simulink model "Katex_FullCar_R2017b_V03"  (R2026a)
settings: Solver=ode1  StopTime=1000  FixedStep=Ts  EnableMultiTasking=on
PostLoadFcn:
  | , if any(exist('dsrtsu_mdlpostloadfcn', 'file') == [2, 3, 6]), try dsrtsu_mdlpostloadfcn('Execute', bdroot); catch fprintf('Error in PostLoadFcn (dsrtsu_mdlpostloadfcn) for model "%s":\n %s\n', bdroot, lasterr); end, end,
  | , if any(exist('dsrtsu_mdlpostloadfcn', 'file') ~= 0), dsrtsu_mdlpostloadfcn('Execute', bdroot); end,
InitFcn:
  | , if any(exist('rtifpga_mdlclblib', 'file') ~= 0), rtifpga_mdlclblib('Init', bdroot); end,
  | 
  | 
  | init
undefined symbols (not defined in the file): locklim_sus, roundN, Ts
libraries: sl_discontinuities x29, simulink_extras x26, simulink x22, mjLib x1
(part 6 of 10)

== system Katex_FullCar_R2017b_V03/DGIST/_High_Level_Ctrl/Chassis_FB_ctrl/Slip control FR/Subsystem/Subsystem1 ==
  In1 : Inport
  Constant2 : Constant
  Constant3 : Constant  Value=-1
  If : If  IfExpression=u1 >= 0  ElseIfExpressions=u1<0
  If Action Subsystem : Subsystem  TreatAsAtomicUnit=on
  If Action Subsystem1 : Subsystem  TreatAsAtomicUnit=on
  Merge : Merge
  sign : Outport  VectorParamsAs1DForOutWhenUnconnected=off
  wires:
  If Action Subsystem/1(Out1) -> Merge/1
  If Action Subsystem1/1(Out1) -> Merge/2
  Constant3/1 -> If Action Subsystem1/1(In1)
  In1/1 -> If/1
  Merge/1 -> sign/1
  Constant2/1 -> If Action Subsystem/1(In1)
  If/2 -> If Action Subsystem1/Action
  If/1 -> If Action Subsystem/Action

== system Katex_FullCar_R2017b_V03/DGIST/_Low_Level_Ctrl/Driving_Low_Level_Controller/Torque Mode/Driving Wheel Control/DOB(omega) ==
  U_in*(Tm) : Inport
  Y_out(w) : Inport  Port=2
  CutoffFreq_Q : Inport  Port=3
  ControlOnOff : Inport  Port=4
  Add1 : Sum  Inputs=-+
  Add2 : Sum  Inputs=+++
  Delay : Delay  DelayLength=1  InitialCondition=0
  Divide{1..2,4..6} (5 alike) : Product  Inputs=**
  Dot2 : Subsystem
      mask Display: disp('dot')
  LPF : Subsystem
  Dist_hat : Outport  VectorParamsAs1DForOutWhenUnconnected=off
  wires:
  Add1/1 -> LPF/1(In)
  CutoffFreq_Q/1 -> LPF/2(fc)
  LPF/1(Out) -> Divide6/1
  Dot2/1(out) -> Divide2/2
  ControlOnOff/1 -> Divide6/2, Divide5/2, Divide1/2
  Y_out(w)/1 -> Divide1/1
  [Local_Bn] -> Divide4/1
  Divide2/1 -> Add2/1
  [Local_Jn] -> Divide2/1
  Divide1/1 -> Divide4/2, Dot2/1(in)
  Divide4/1 -> Add2/2
  Add2/1 -> Add1/2
  U_in*(Tm)/1 -> Delay/1
  Divide5/1 -> Add1/1
  Divide6/1 -> Dist_hat/1
  [wheel_Bn] -> [Local_Bn]
  [wheel_Jn] -> [Local_Jn]
  Delay/1 -> Divide5/1

== system Katex_FullCar_R2017b_V03/DGIST/_Low_Level_Ctrl/Driving_Low_Level_Controller/Torque Mode/Driving Wheel Control/Feedforward(omega) ==
  command : Inport
  LFP cutoff : Inport  Port=2
  ControlOnOff : Inport  Port=3
  Add5 : Sum  Inputs=+++
  Divide{,1..2,4} (4 alike) : Product  Inputs=**
  Dot2 : Subsystem
      mask Display: disp('dot')
  LPF : Subsystem
  FF : Outport  VectorParamsAs1DForOutWhenUnconnected=off
  wires:
  LFP cutoff/1 -> LPF/2(fc)
  Add5/1 -> LPF/1(In)
  LPF/1(Out) -> Divide/1
  Divide/1 -> FF/1
  ControlOnOff/1 -> Divide1/2, Divide/2
  Divide1/1 -> Divide4/2, Dot2/1(in)
  [wheel_Jn] -> [Local_Jn]
  [wheel_Bn] -> [Local_Bn]
  command/1 -> Divide1/1
  Divide2/1 -> Add5/1
  Dot2/1(out) -> Divide2/2
  [Local_Jn] -> Divide2/1
  Divide4/1 -> Add5/2
  [Local_Bn] -> Divide4/1

== system Katex_FullCar_R2017b_V03/DGIST/_Low_Level_Ctrl/Driving_Low_Level_Controller/Torque Mode/Driving Wheel Control/Poleplacement(PI)1 ==
  note: H(s) = (Kp+Ki)/(s)
  error : Inport
  BW : Inport  Port=2
  zeta : Inport  Port=3
  ConstrolOnOff : Inport  Port=4
  ControlInputError : Inport  Port=5
  Add : Sum
  Add1 : Sum  Inputs=+-
  Constant1 : Constant  Value=Ts
  Divide{,1..5,7} (7 alike) : Product  Inputs=**
  Divide6 : Product  Inputs=***
  Divide9 : Product  Inputs=**/
  Integrator1 : Subsystem
      mask Display: disp('Integator')
  Saturation : Saturate  UpperLimit=3  LowerLimit=0.5
  Saturation Dynamic : sl_discontinuities/Saturation Dynamic  OutMin=[]  OutMax=[]  OutDataTypeStr=Inherit: Same as second input  OutDataType=fixdt(1, 16)  OutScaling=2^-10  DoSatur=off
  Sum1 : Sum  Inputs=|++
  Sum2 : Sum  Inputs=++|
  "gain " : Gain  Gain=2*pi
  gain 1 : Gain  Gain=2
  feedback gain : Outport  VectorParamsAs1DForOutWhenUnconnected=off
  wires:
  BW/1 -> "gain "/1
  zeta/1 -> Saturation/1
  Saturation/1 -> gain 1/1
  [Local_Bn] -> Add1/2
  Divide1/1 -> Sum1/1
  Divide2/1 -> Sum1/2
  Integrator1/1(out) -> Divide2/1
  gain 1/1 -> Divide6/1
  Divide3/1 -> Divide4/1
  [wheel_Bn] -> [Local_Bn]
  [wheel_Jn] -> [Local_Jn]
  [Local_Jn] -> Divide4/2
  [Local_Jn] -> Divide6/3
  Divide6/1 -> Add1/1
  Add1/1 -> [Kp]
  Divide4/1 -> [Ki]
  [Kp] -> Divide1/1
  error/1 -> Divide/1
  Sum1/1 -> Divide5/1
  Divide5/1 -> feedback gain/1
  ConstrolOnOff/1 -> Divide5/2, Integrator1/2("Off : 0 On : 1"), Divide/2
  [Ki] -> Divide2/2
  ControlInputError/1 -> Divide7/1
  Divide/1 -> Divide1/2, Sum2/1
  Sum2/1 -> Integrator1/1(in)
  Divide7/1 -> Sum2/2
  Add/1 -> Saturation Dynamic/1
  Divide9/1 -> [AntiWindup]
  Constant1/1 -> Saturation Dynamic/3
  "gain "/1 -> Divide9/2, Add/1, Divide9/1, Divide6/2, Divide3/1, Divide3/2
  [Ki] -> Add/2, Saturation Dynamic/2
  [AntiWindup] -> Divide7/2
  Saturation Dynamic/1 -> Divide9/3

== system Katex_FullCar_R2017b_V03/DGIST/_Low_Level_Ctrl/Driving_Low_Level_Controller/Torque Mode/Driving Wheel Control/Subsystem ==
  note: wheel N*m
  note: mN*m
  note: Motor N*m
  N*m : Inport
  Constant1 : Constant  Value=1000
  Divide : Product  Inputs=*/
  Divide1 : Product  Inputs=**
  Divide3 : Product  Inputs=*/
  Gain : Gain  Gain=1000
  Gain1 : Gain  Gain=-1
  Saturation Dynamic : sl_discontinuities/Saturation Dynamic  OutMin=[]  OutMax=[]  OutDataTypeStr=Inherit: Same as second input  OutDataType=fixdt(1, 16)  OutScaling=2^-10  DoSatur=off
  Target Torque : Outport  VectorParamsAs1DForOutWhenUnconnected=off
  wires:
  [N_dri] -> Divide3/2
  Gain/1 -> Target Torque/1
  Divide/1 -> Gain/1
  N*m/1 -> Divide3/1
  Divide1/1 -> Saturation Dynamic/2
  Constant1/1 -> Divide1/2
  Divide3/1 -> Divide1/1
  Saturation Dynamic/1 -> Divide/1
  Gain1/1 -> Saturation Dynamic/3
  [Dri_rated_torque] -> Saturation Dynamic/1, Gain1/1, Divide/2

== system Katex_FullCar_R2017b_V03/DGIST/_Low_Level_Ctrl/Steering_Low_Level_Controller/Torque Mode/Steering Motor Control/DOB(omega) ==
  U_in*(Tm) : Inport
  Y_out(w) : Inport  Port=2
  CutoffFreq_Q : Inport  Port=3
  ControlOnOff : Inport  Port=4
  Add1 : Sum  Inputs=-+
  Add2 : Sum  Inputs=+++
  Delay : Delay  DelayLength=1  InitialCondition=0
  Divide{1..2,4..6} (5 alike) : Product  Inputs=**
  Dot2 : Subsystem
      mask Display: disp('dot')
  LPF : Subsystem
  Dist_hat : Outport  VectorParamsAs1DForOutWhenUnconnected=off
  wires:
  Add1/1 -> LPF/1(In)
  CutoffFreq_Q/1 -> LPF/2(fc)
  LPF/1(Out) -> Divide6/1
  Dot2/1(out) -> Divide2/2
  ControlOnOff/1 -> Divide6/2, Divide5/2, Divide1/2
  Y_out(w)/1 -> Divide1/1
  [Local_Bn] -> Divide4/1
  Divide2/1 -> Add2/1
  [Local_Jn] -> Divide2/1
  Divide1/1 -> Divide4/2, Dot2/1(in)
  Divide4/1 -> Add2/2
  Add2/1 -> Add1/2
  U_in*(Tm)/1 -> Delay/1
  Divide5/1 -> Add1/1
  Divide6/1 -> Dist_hat/1
  [steer_Bn] -> [Local_Bn]
  [steer_Jn] -> [Local_Jn]
  Delay/1 -> Divide5/1

== system Katex_FullCar_R2017b_V03/DGIST/_Low_Level_Ctrl/Steering_Low_Level_Controller/Torque Mode/Steering Motor Control/DOB(theta) ==
  U_in*(Tm) : Inport
  Y_out(theta) : Inport  Port=2
  CutoffFreq_Q : Inport  Port=3
  ConstrolOnOff : Inport  Port=4
  Add1 : Sum  Inputs=-+
  Add5 : Sum  Inputs=+++
  Delay : Delay  DelayLength=1  InitialCondition=0
  Divide{,1..5} (6 alike) : Product  Inputs=**
  Dot : Subsystem
      mask Display: disp('dot')
  Dot1 : Subsystem
      mask Display: disp('dot')
  Dot2 : Subsystem
      mask Display: disp('dot')
  NominalModel_Kn : Constant  Value=0
  Scope1 : Scope
  Scope2 : Scope
      settings: DataLoggingVariableName=ScopeData2
  Scope3 : Scope
      settings: DataLoggingVariableName=ScopeData3
  Second order LPF : Subsystem
  zeta : Constant  SampleTime=Ts
  Dist_hat : Outport  VectorParamsAs1DForOutWhenUnconnected=off
  wires:
  Add5/1 -> Add1/2
  CutoffFreq_Q/1 -> Second order LPF/2(fc)
  zeta/1 -> Second order LPF/3(zeta)
  [steer_Jn] -> [Local_Jn]
  NominalModel_Kn/1 -> [Local_Kn]
  [steer_Bn] -> [Local_Bn]
  Y_out(theta)/1 -> Scope1/1, Divide4/1
  [Local_Jn] -> Divide/2
  [Local_Kn] -> Divide2/2
  Dot1/1(out) -> Divide1/1
  [Local_Bn] -> Divide1/2
  Dot/1(out) -> Dot2/1(in)
  Divide/1 -> Add5/1
  Divide2/1 -> Add5/3
  Divide1/1 -> Add5/2
  Dot2/1(out) -> Divide/1
  ConstrolOnOff/1 -> Divide5/2, Divide3/2, Divide4/2
  Divide4/1 -> Divide2/1, Dot1/1(in), Dot/1(in)
  U_in*(Tm)/1 -> Delay/1
  Divide3/1 -> Add1/1
  Second order LPF/1(Dist_hat) -> Divide5/1
  Divide5/1 -> Scope2/1, Dist_hat/1
  Delay/1 -> Divide3/1
  Add1/1 -> Scope3/1, Second order LPF/1(In)

== system Katex_FullCar_R2017b_V03/DGIST/_Low_Level_Ctrl/Steering_Low_Level_Controller/Torque Mode/Steering Motor Control/Feedforward(omega) ==
  command : Inport
  LFP cutoff : Inport  Port=2
  ControlOnOff : Inport  Port=3
  Add5 : Sum  Inputs=+++
  Divide{,1..2,4} (4 alike) : Product  Inputs=**
  Dot2 : Subsystem
      mask Display: disp('dot')
  LPF : Subsystem
  FF : Outport  VectorParamsAs1DForOutWhenUnconnected=off
  wires:
  LFP cutoff/1 -> LPF/2(fc)
  Add5/1 -> LPF/1(In)
  LPF/1(Out) -> Divide/1
  Divide/1 -> FF/1
  ControlOnOff/1 -> Divide/2, Divide1/2
  Divide1/1 -> Divide4/2, Dot2/1(in)
  [steer_Jn] -> [Local_Jn]
  [steer_Bn] -> [Local_Bn]
  command/1 -> Divide1/1
  Divide2/1 -> Add5/1
  Dot2/1(out) -> Divide2/2
  [Local_Jn] -> Divide2/1
  Divide4/1 -> Add5/2
  [Local_Bn] -> Divide4/1

== system Katex_FullCar_R2017b_V03/DGIST/_Low_Level_Ctrl/Steering_Low_Level_Controller/Torque Mode/Steering Motor Control/Feedforward(theta) ==
  command : Inport
  LFP cutoff : Inport  Port=2
  LPF zeta : Inport  Port=3
  ConstrolOnOff : Inport  Port=4
  Add5 : Sum  Inputs=+++
  Divide{,1..4} (5 alike) : Product  Inputs=**
  Dot : Subsystem
      mask Display: disp('dot')
  Dot1 : Subsystem
      mask Display: disp('dot')
  Dot2 : Subsystem
      mask Display: disp('dot')
  NominalModel_Kn : Constant  Value=0
  Scope : Scope
      settings: ActiveDisplayYMinimum=-1  ActiveDisplayYMaximum=1  DataLoggingVariableName=ScopeData2
  Scope1 : Scope
      settings: ActiveDisplayYMinimum=-1  ActiveDisplayYMaximum=1  DataLoggingVariableName=ScopeData5
  Second order LPF : Subsystem
  before_dot : Scope
      settings: DataLoggingVariableName=ScopeData3
  commad : Scope
      settings: DataLoggingVariableName=ScopeData4
  FF : Outport  VectorParamsAs1DForOutWhenUnconnected=off
  wires:
  Dot/1(out) -> Dot2/1(in)
  Dot1/1(out) -> Divide1/1
  LFP cutoff/1 -> Second order LPF/2(fc)
  Dot2/1(out) -> Divide/1
  Add5/1 -> Second order LPF/1(In)
  LPF zeta/1 -> Second order LPF/3(zeta)
  Divide/1 -> Scope/1, Add5/1
  Divide1/1 -> Scope1/1, Add5/2
  Divide2/1 -> Add5/3
  [Local_Jn] -> Divide/2
  [Local_Bn] -> Divide1/2
  [Local_Kn] -> Divide2/2
  [steer_Jn] -> [Local_Jn]
  [steer_Bn] -> [Local_Bn]
  NominalModel_Kn/1 -> [Local_Kn]
  Second order LPF/1(Out) -> Divide3/1
  Divide3/1 -> FF/1
  ConstrolOnOff/1 -> Divide4/2, Divide3/2
  Divide4/1 -> Divide2/1, Dot1/1(in), before_dot/1, Dot/1(in)
  command/1 -> commad/1, Divide4/1

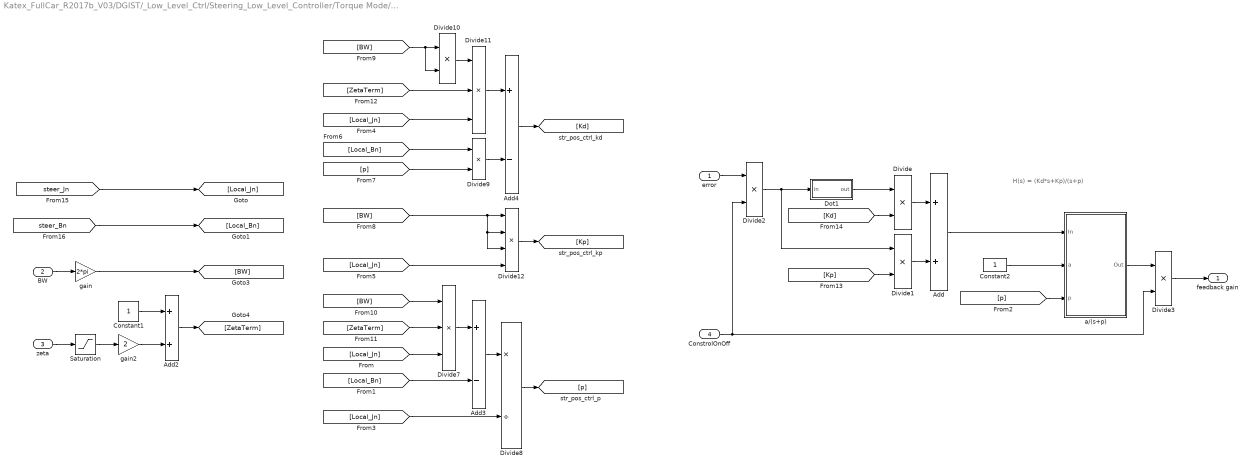
== system Katex_FullCar_R2017b_V03/DGIST/_Low_Level_Ctrl/Steering_Low_Level_Controller/Torque Mode/Steering Motor Control/Lag compensator(zeta) ==
  note: H(s) = (Kd*s+Kp)/(s+p)
  error : Inport
  BW : Inport  Port=2
  zeta : Inport  Port=3
  ConstrolOnOff : Inport  Port=4
  Add : Sum
  Add2 : Sum
  Add3 : Sum  Inputs=+-
  Add4 : Sum  Inputs=+-
  Constant1 : Constant  SampleTime=Ts
  Constant2 : Constant  SampleTime=Ts
  Divide{,1..3,9..10} (6 alike) : Product  Inputs=**
  Divide11 : Product  Inputs=***
  Divide12 : Product  Inputs=****
  Divide7 : Product  Inputs=***
  Divide8 : Product  Inputs=*/
  Dot1 : Subsystem
      mask Display: disp('dot')
  Saturation : Saturate  UpperLimit=1.5  LowerLimit=0.5
  a/(s+p) : Subsystem
  "gain " : Gain  Gain=2*pi
  gain2 : Gain  Gain=2
  feedback gain : Outport  VectorParamsAs1DForOutWhenUnconnected=off
  wires:
  BW/1 -> "gain "/1
  Add/1 -> a/(s+p)/1(In)
  Divide/1 -> Add/1
  Dot1/1(out) -> Divide/1
  Constant2/1 -> a/(s+p)/2(a)
  zeta/1 -> Saturation/1
  Saturation/1 -> gain2/1
  gain2/1 -> Add2/2
  Constant1/1 -> Add2/1
  [Local_Jn] -> Divide7/3
  Divide7/1 -> Add3/1
  [Local_Bn] -> Add3/2
  Add3/1 -> Divide8/1
  Divide10/1 -> Divide11/1
  Divide8/1 -> [p]
  Divide9/1 -> Add4/2
  Divide11/1 -> Add4/1
  [p] -> a/(s+p)/3(p)
  Divide1/1 -> Add/2
  [Local_Jn] -> Divide8/2
  [Local_Jn] -> Divide11/3
  [Local_Jn] -> Divide12/4
  [Local_Bn] -> Divide9/1
  [p] -> Divide9/2
  "gain "/1 -> [BW]
  [BW] -> Divide12/3, Divide12/2, Divide12/1
  [BW] -> Divide10/2, Divide10/1
  [BW] -> Divide7/1
  Add2/1 -> [ZetaTerm]
  [ZetaTerm] -> Divide7/2
  [ZetaTerm] -> Divide11/2
  Add4/1 -> [Kd]
  Divide12/1 -> [Kp]
  [Kp] -> Divide1/2
  [Kd] -> Divide/2
  [steer_Jn] -> [Local_Jn]
  [steer_Bn] -> [Local_Bn]
  error/1 -> Divide2/1
  Divide2/1 -> Divide1/1, Dot1/1(in)
  ConstrolOnOff/1 -> Divide3/2, Divide2/2
  a/(s+p)/1(Out) -> Divide3/1
  Divide3/1 -> feedback gain/1

== system Katex_FullCar_R2017b_V03/DGIST/_Low_Level_Ctrl/Steering_Low_Level_Controller/Torque Mode/Steering Motor Control/Poleplacement(PI)1 ==
  note: H(s) = (Kp+Ki)/(s)
  error : Inport
  BW : Inport  Port=2
  zeta : Inport  Port=3
  ConstrolOnOff : Inport  Port=4
  ControlInputError : Inport  Port=5
  Add : Sum
  Add1 : Sum  Inputs=+-
  Constant1 : Constant  Value=Ts
  Divide{,1..5,7} (7 alike) : Product  Inputs=**
  Divide6 : Product  Inputs=***
  Divide9 : Product  Inputs=**/
  Integrator1 : Subsystem
      mask Display: disp('Integator')
  Saturation : Saturate  UpperLimit=3  LowerLimit=0.5
  Saturation Dynamic : simulink/Discontinuities/Saturation Dynamic  OutMin=[]  OutMax=[]  OutDataTypeStr=Inherit: Same as second input  OutDataType=fixdt(1, 16)  OutScaling=2^-10  DoSatur=off
  Sum1 : Sum  Inputs=|++
  Sum2 : Sum  Inputs=++|
  "gain " : Gain  Gain=2*pi
  gain 1 : Gain  Gain=2
  feedback gain : Outport  VectorParamsAs1DForOutWhenUnconnected=off
  wires:
  BW/1 -> "gain "/1
  zeta/1 -> Saturation/1
  Saturation/1 -> gain 1/1
  [Local_Bn] -> Add1/2
  Divide1/1 -> Sum1/1
  Divide2/1 -> Sum1/2
  Integrator1/1(out) -> Divide2/1
  gain 1/1 -> Divide6/1
  Divide3/1 -> Divide4/1
  [Local_Jn] -> Divide4/2
  [Local_Jn] -> Divide6/3
  Divide6/1 -> Add1/1
  Add1/1 -> [Kp]
  Divide4/1 -> [Ki]
  [Kp] -> Divide1/1
  error/1 -> Divide/1
  Sum1/1 -> Divide5/1
  Divide5/1 -> feedback gain/1
  ConstrolOnOff/1 -> Divide5/2, Integrator1/2("Off : 0 On : 1"), Divide/2
  [Ki] -> Divide2/2
  ControlInputError/1 -> Divide7/1
  Divide/1 -> Divide1/2, Sum2/1
  Sum2/1 -> Integrator1/1(in)
  Divide7/1 -> Sum2/2
  Add/1 -> Saturation Dynamic/1
  Divide9/1 -> [AntiWindup]
  Constant1/1 -> Saturation Dynamic/3
  "gain "/1 -> Divide9/2, Add/1, Divide9/1, Divide6/2, Divide3/1, Divide3/2
  [Ki] -> Add/2, Saturation Dynamic/2
  [AntiWindup] -> Divide7/2
  Saturation Dynamic/1 -> Divide9/3
  [steer_Jn] -> [Local_Jn]
  [steer_Bn] -> [Local_Bn]

== system Katex_FullCar_R2017b_V03/DGIST/_Low_Level_Ctrl/Steering_Low_Level_Controller/Torque Mode/Steering Motor Control/Steering Ref Mode  ==
  Constant2 : Constant  Value=0
  If : If  IfExpression=u1 == 0  ElseIfExpressions=u1 ==1
  If Action Subsystem : Subsystem  TreatAsAtomicUnit=on
  If Action Subsystem1 : Subsystem  TreatAsAtomicUnit=on
  If Action Subsystem2 : Subsystem  TreatAsAtomicUnit=on
  Merge : Merge  Inputs=3
  Out1 : Outport  VectorParamsAs1DForOutWhenUnconnected=off
  wires:
  Constant2/1 -> If Action Subsystem/1(In1)
  [sine_ref] -> If Action Subsystem1/1(In1)
  Merge/1 -> Out1/1
  If Action Subsystem/1(Out1) -> Merge/1
  If Action Subsystem2/1(Out1) -> Merge/3
  [str_load_target_pos] -> If Action Subsystem2/1(In1)
  If Action Subsystem1/1(Out1) -> Merge/2
  If/2 -> If Action Subsystem1/Action
  If/3 -> If Action Subsystem2/Action
  [str_ref_mode] -> If/1
  If/1 -> If Action Subsystem/Action

== system Katex_FullCar_R2017b_V03/DGIST/_Low_Level_Ctrl/Steering_Low_Level_Controller/Torque Mode/Steering Motor Control/Steering system ==
  note: mN*m
  note: Motor N*m
  note: Load N*m
  N*m : Inport
  Constant : Constant  Value=55.08
  Constant1 : Constant  Value=1000
  Constant2 : Constant  Value=315
  Divide : Product  Inputs=*/
  Divide1 : Product  Inputs=**
  Divide3 : Product  Inputs=*/
  Gain : Gain  Gain=1000
  Gain1 : Gain  Gain=-1
  Saturation Dynamic : simulink/Discontinuities/Saturation Dynamic  OutMin=[]  OutMax=[]  OutDataTypeStr=Inherit: Same as second input  OutDataType=fixdt(1, 16)  OutScaling=2^-10  DoSatur=off
  Target Torque : Outport  VectorParamsAs1DForOutWhenUnconnected=off
  tag scope: closed_ID_FB=global
  wires:
  Constant2/1 -> Divide3/2
  Gain/1 -> Target Torque/1
  Divide/1 -> Gain/1
  N*m/1 -> Divide3/1
  Divide1/1 -> [closed_ID_FB], Saturation Dynamic/2
  Constant1/1 -> Divide1/2
  Divide3/1 -> Divide1/1
  Saturation Dynamic/1 -> Divide/1
  Gain1/1 -> Saturation Dynamic/3
  Constant/1 -> Saturation Dynamic/1, Gain1/1, Divide/2

== system Katex_FullCar_R2017b_V03/DGIST/_Low_Level_Ctrl/Steering_Low_Level_Controller/Torque Mode/Steering Motor Control/Steering system1 ==
  note: mN*m
  note: Motor N*m
  note: Load N*m
  N*m : Inport
  Constant1 : Constant  Value=1000
  Constant2 : Constant  Value=315
  Divide : Product  Inputs=*/
  Divide1 : Product  Inputs=**
  Divide3 : Product  Inputs=*/
  Gain : Gain  Gain=1000
  Gain1 : Gain  Gain=-1
  Saturation Dynamic : sl_discontinuities/Saturation Dynamic  OutMin=[]  OutMax=[]  OutDataTypeStr=Inherit: Same as second input  OutDataType=fixdt(1, 16)  OutScaling=2^-10  DoSatur=off
  Target Torque : Outport  VectorParamsAs1DForOutWhenUnconnected=off
  wires:
  Constant2/1 -> Divide3/2
  Gain/1 -> Target Torque/1
  Divide/1 -> Gain/1
  N*m/1 -> Divide3/1
  Divide1/1 -> Saturation Dynamic/2
  Constant1/1 -> Divide1/2
  Divide3/1 -> Divide1/1
  Saturation Dynamic/1 -> Divide/1
  Gain1/1 -> Saturation Dynamic/3
  [str_rated_torque] -> Saturation Dynamic/1, Gain1/1, Divide/2

== system Katex_FullCar_R2017b_V03/DGIST/_Low_Level_Ctrl/Steering_Low_Level_Controller/Torque Mode/Steering Motor Control1/DOB(theta) ==
  U_in*(Tm) : Inport
  Y_out(theta) : Inport  Port=2
  CutoffFreq_Q : Inport  Port=3
  ConstrolOnOff : Inport  Port=4
  Add1 : Sum  Inputs=-+
  Add5 : Sum  Inputs=+++
  Delay : Delay  DelayLength=1  InitialCondition=0
  Divide{,1..5} (6 alike) : Product  Inputs=**
  Dot : Subsystem
      mask Display: disp('dot')
  Dot1 : Subsystem
      mask Display: disp('dot')
  Dot2 : Subsystem
      mask Display: disp('dot')
  NominalModel_Kn : Constant  Value=0
  Scope1 : Scope
  Scope2 : Scope
      settings: DataLoggingVariableName=ScopeData2
  Scope3 : Scope
      settings: DataLoggingVariableName=ScopeData3
  Second order LPF : Subsystem
  zeta : Constant  SampleTime=Ts
  Dist_hat : Outport  VectorParamsAs1DForOutWhenUnconnected=off
  wires:
  Add5/1 -> Add1/2
  CutoffFreq_Q/1 -> Second order LPF/2(fc)
  zeta/1 -> Second order LPF/3(zeta)
  [steer_Jn] -> [Local_Jn]
  NominalModel_Kn/1 -> [Local_Kn]
  [steer_Bn] -> [Local_Bn]
  Y_out(theta)/1 -> Scope1/1, Divide4/1
  [Local_Jn] -> Divide/2
  [Local_Kn] -> Divide2/2
  Dot1/1(out) -> Divide1/1
  [Local_Bn] -> Divide1/2
  Dot/1(out) -> Dot2/1(in)
  Divide/1 -> Add5/1
  Divide2/1 -> Add5/3
  Divide1/1 -> Add5/2
  Dot2/1(out) -> Divide/1
  ConstrolOnOff/1 -> Divide5/2, Divide3/2, Divide4/2
  Divide4/1 -> Divide2/1, Dot1/1(in), Dot/1(in)
  U_in*(Tm)/1 -> Delay/1
  Divide3/1 -> Add1/1
  Second order LPF/1(Dist_hat) -> Divide5/1
  Divide5/1 -> Scope2/1, Dist_hat/1
  Delay/1 -> Divide3/1
  Add1/1 -> Scope3/1, Second order LPF/1(In)

== system Katex_FullCar_R2017b_V03/DGIST/_Low_Level_Ctrl/Steering_Low_Level_Controller/Torque Mode/Steering Motor Control1/Feedforward(theta) ==
  command : Inport
  LFP cutoff : Inport  Port=2
  LPF zeta : Inport  Port=3
  ConstrolOnOff : Inport  Port=4
  Add5 : Sum  Inputs=+++
  Divide{,1..4} (5 alike) : Product  Inputs=**
  Dot : Subsystem
      mask Display: disp('dot')
  Dot1 : Subsystem
      mask Display: disp('dot')
  Dot2 : Subsystem
      mask Display: disp('dot')
  NominalModel_Kn : Constant  Value=0
  Scope : Scope
      settings: ActiveDisplayYMinimum=-1  ActiveDisplayYMaximum=1  DataLoggingVariableName=ScopeData2
  Scope1 : Scope
      settings: ActiveDisplayYMinimum=-1  ActiveDisplayYMaximum=1  DataLoggingVariableName=ScopeData5
  Second order LPF : Subsystem
  before_dot : Scope
      settings: DataLoggingVariableName=ScopeData3
  commad : Scope
      settings: DataLoggingVariableName=ScopeData4
  FF : Outport  VectorParamsAs1DForOutWhenUnconnected=off
  wires:
  Dot/1(out) -> Dot2/1(in)
  Dot1/1(out) -> Divide1/1
  LFP cutoff/1 -> Second order LPF/2(fc)
  Dot2/1(out) -> Divide/1
  Add5/1 -> Second order LPF/1(In)
  LPF zeta/1 -> Second order LPF/3(zeta)
  Divide/1 -> Scope/1, Add5/1
  Divide1/1 -> Scope1/1, Add5/2
  Divide2/1 -> Add5/3
  [Local_Jn] -> Divide/2
  [Local_Bn] -> Divide1/2
  [Local_Kn] -> Divide2/2
  [steer_Jn] -> [Local_Jn]
  [steer_Bn] -> [Local_Bn]
  NominalModel_Kn/1 -> [Local_Kn]
  Second order LPF/1(Out) -> Divide3/1
  Divide3/1 -> FF/1
  ConstrolOnOff/1 -> Divide4/2, Divide3/2
  Divide4/1 -> Divide2/1, Dot1/1(in), before_dot/1, Dot/1(in)
  command/1 -> commad/1, Divide4/1

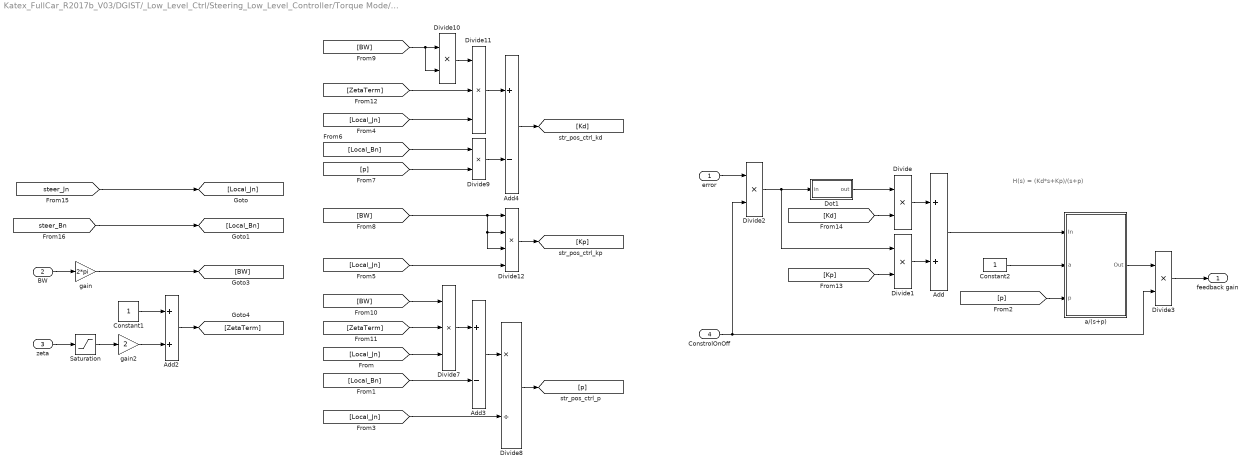
== system Katex_FullCar_R2017b_V03/DGIST/_Low_Level_Ctrl/Steering_Low_Level_Controller/Torque Mode/Steering Motor Control1/Lag compensator(zeta) ==
  note: H(s) = (Kd*s+Kp)/(s+p)
  error : Inport
  BW : Inport  Port=2
  zeta : Inport  Port=3
  ConstrolOnOff : Inport  Port=4
  Add : Sum
  Add2 : Sum
  Add3 : Sum  Inputs=+-
  Add4 : Sum  Inputs=+-
  Constant1 : Constant  SampleTime=Ts
  Constant2 : Constant  SampleTime=Ts
  Divide{,1..3,9..10} (6 alike) : Product  Inputs=**
  Divide11 : Product  Inputs=***
  Divide12 : Product  Inputs=****
  Divide7 : Product  Inputs=***
  Divide8 : Product  Inputs=*/
  Dot1 : Subsystem
      mask Display: disp('dot')
  Saturation : Saturate  UpperLimit=1.5  LowerLimit=0.5
  a/(s+p) : Subsystem
  "gain " : Gain  Gain=2*pi
  gain2 : Gain  Gain=2
  feedback gain : Outport  VectorParamsAs1DForOutWhenUnconnected=off
  wires:
  BW/1 -> "gain "/1
  Add/1 -> a/(s+p)/1(In)
  Divide/1 -> Add/1
  Dot1/1(out) -> Divide/1
  Constant2/1 -> a/(s+p)/2(a)
  zeta/1 -> Saturation/1
  Saturation/1 -> gain2/1
  gain2/1 -> Add2/2
  Constant1/1 -> Add2/1
  [Local_Jn] -> Divide7/3
  Divide7/1 -> Add3/1
  [Local_Bn] -> Add3/2
  Add3/1 -> Divide8/1
  Divide10/1 -> Divide11/1
  Divide8/1 -> [p]
  Divide9/1 -> Add4/2
  Divide11/1 -> Add4/1
  [p] -> a/(s+p)/3(p)
  Divide1/1 -> Add/2
  [Local_Jn] -> Divide8/2
  [Local_Jn] -> Divide11/3
  [Local_Jn] -> Divide12/4
  [Local_Bn] -> Divide9/1
  [p] -> Divide9/2
  "gain "/1 -> [BW]
  [BW] -> Divide12/3, Divide12/2, Divide12/1
  [BW] -> Divide10/2, Divide10/1
  [BW] -> Divide7/1
  Add2/1 -> [ZetaTerm]
  [ZetaTerm] -> Divide7/2
  [ZetaTerm] -> Divide11/2
  Add4/1 -> [Kd]
  Divide12/1 -> [Kp]
  [Kp] -> Divide1/2
  [Kd] -> Divide/2
  [steer_Jn] -> [Local_Jn]
  [steer_Bn] -> [Local_Bn]
  error/1 -> Divide2/1
  Divide2/1 -> Divide1/1, Dot1/1(in)
  ConstrolOnOff/1 -> Divide3/2, Divide2/2
  a/(s+p)/1(Out) -> Divide3/1
  Divide3/1 -> feedback gain/1

== system Katex_FullCar_R2017b_V03/DGIST/_Low_Level_Ctrl/Steering_Low_Level_Controller/Torque Mode/Steering Motor Control1/Steering system1 ==
  note: mN*m
  note: Motor N*m
  note: Load N*m
  N*m : Inport
  Constant1 : Constant  Value=1000
  Constant2 : Constant  Value=315
  Divide : Product  Inputs=*/
  Divide1 : Product  Inputs=**
  Divide3 : Product  Inputs=*/
  Gain : Gain  Gain=1000
  Gain1 : Gain  Gain=-1
  Saturation Dynamic : sl_discontinuities/Saturation Dynamic  OutMin=[]  OutMax=[]  OutDataTypeStr=Inherit: Same as second input  OutDataType=fixdt(1, 16)  OutScaling=2^-10  DoSatur=off
  Target Torque : Outport  VectorParamsAs1DForOutWhenUnconnected=off
  wires:
  Constant2/1 -> Divide3/2
  Gain/1 -> Target Torque/1
  Divide/1 -> Gain/1
  N*m/1 -> Divide3/1
  Divide1/1 -> Saturation Dynamic/2
  Constant1/1 -> Divide1/2
  Divide3/1 -> Divide1/1
  Saturation Dynamic/1 -> Divide/1
  Gain1/1 -> Saturation Dynamic/3
  [str_rated_torque] -> Saturation Dynamic/1, Gain1/1, Divide/2

== system Katex_FullCar_R2017b_V03/DGIST/_Low_Level_Ctrl/Steering_Low_Level_Controller/Torque Mode/Steering Motor Control2/DOB(omega) ==
  U_in*(Tm) : Inport
  Y_out(w) : Inport  Port=2
  CutoffFreq_Q : Inport  Port=3
  ControlOnOff : Inport  Port=4
  Add1 : Sum  Inputs=-+
  Add2 : Sum  Inputs=+++
  Delay : Delay  DelayLength=1  InitialCondition=0
  Divide{1..2,4..6} (5 alike) : Product  Inputs=**
  Dot2 : Subsystem
      mask Display: disp('dot')
  LPF : Subsystem
  Dist_hat : Outport  VectorParamsAs1DForOutWhenUnconnected=off
  wires:
  Add1/1 -> LPF/1(In)
  CutoffFreq_Q/1 -> LPF/2(fc)
  LPF/1(Out) -> Divide6/1
  Dot2/1(out) -> Divide2/2
  ControlOnOff/1 -> Divide6/2, Divide5/2, Divide1/2
  Y_out(w)/1 -> Divide1/1
  [Local_Bn] -> Divide4/1
  Divide2/1 -> Add2/1
  [Local_Jn] -> Divide2/1
  Divide1/1 -> Divide4/2, Dot2/1(in)
  Divide4/1 -> Add2/2
  Add2/1 -> Add1/2
  U_in*(Tm)/1 -> Delay/1
  Divide5/1 -> Add1/1
  Divide6/1 -> Dist_hat/1
  [steer_Bn] -> [Local_Bn]
  [steer_Jn] -> [Local_Jn]
  Delay/1 -> Divide5/1

== system Katex_FullCar_R2017b_V03/DGIST/_Low_Level_Ctrl/Steering_Low_Level_Controller/Torque Mode/Steering Motor Control2/DOB(theta) ==
  U_in*(Tm) : Inport
  Y_out(theta) : Inport  Port=2
  CutoffFreq_Q : Inport  Port=3
  ConstrolOnOff : Inport  Port=4
  Add1 : Sum  Inputs=-+
  Add5 : Sum  Inputs=+++
  Delay : Delay  DelayLength=1  InitialCondition=0
  Divide{,1..5} (6 alike) : Product  Inputs=**
  Dot : Subsystem
      mask Display: disp('dot')
  Dot1 : Subsystem
      mask Display: disp('dot')
  Dot2 : Subsystem
      mask Display: disp('dot')
  NominalModel_Kn : Constant  Value=0
  Scope1 : Scope
  Scope2 : Scope
      settings: DataLoggingVariableName=ScopeData2
  Scope3 : Scope
      settings: DataLoggingVariableName=ScopeData3
  Second order LPF : Subsystem
  zeta : Constant  SampleTime=Ts
  Dist_hat : Outport  VectorParamsAs1DForOutWhenUnconnected=off
  wires:
  Add5/1 -> Add1/2
  CutoffFreq_Q/1 -> Second order LPF/2(fc)
  zeta/1 -> Second order LPF/3(zeta)
  [steer_Jn] -> [Local_Jn]
  NominalModel_Kn/1 -> [Local_Kn]
  [steer_Bn] -> [Local_Bn]
  Y_out(theta)/1 -> Scope1/1, Divide4/1
  [Local_Jn] -> Divide/2
  [Local_Kn] -> Divide2/2
  Dot1/1(out) -> Divide1/1
  [Local_Bn] -> Divide1/2
  Dot/1(out) -> Dot2/1(in)
  Divide/1 -> Add5/1
  Divide2/1 -> Add5/3
  Divide1/1 -> Add5/2
  Dot2/1(out) -> Divide/1
  ConstrolOnOff/1 -> Divide5/2, Divide3/2, Divide4/2
  Divide4/1 -> Divide2/1, Dot1/1(in), Dot/1(in)
  U_in*(Tm)/1 -> Delay/1
  Divide3/1 -> Add1/1
  Second order LPF/1(Dist_hat) -> Divide5/1
  Divide5/1 -> Scope2/1, Dist_hat/1
  Delay/1 -> Divide3/1
  Add1/1 -> Scope3/1, Second order LPF/1(In)

== system Katex_FullCar_R2017b_V03/DGIST/_Low_Level_Ctrl/Steering_Low_Level_Controller/Torque Mode/Steering Motor Control2/Feedforward(omega) ==
  command : Inport
  LFP cutoff : Inport  Port=2
  ControlOnOff : Inport  Port=3
  Add5 : Sum  Inputs=+++
  Divide{,1..2,4} (4 alike) : Product  Inputs=**
  Dot2 : Subsystem
      mask Display: disp('dot')
  LPF : Subsystem
  FF : Outport  VectorParamsAs1DForOutWhenUnconnected=off
  wires:
  LFP cutoff/1 -> LPF/2(fc)
  Add5/1 -> LPF/1(In)
  LPF/1(Out) -> Divide/1
  Divide/1 -> FF/1
  ControlOnOff/1 -> Divide/2, Divide1/2
  Divide1/1 -> Divide4/2, Dot2/1(in)
  [steer_Jn] -> [Local_Jn]
  [steer_Bn] -> [Local_Bn]
  command/1 -> Divide1/1
  Divide2/1 -> Add5/1
  Dot2/1(out) -> Divide2/2
  [Local_Jn] -> Divide2/1
  Divide4/1 -> Add5/2
  [Local_Bn] -> Divide4/1

== system Katex_FullCar_R2017b_V03/DGIST/_Low_Level_Ctrl/Steering_Low_Level_Controller/Torque Mode/Steering Motor Control2/Feedforward(theta) ==
  command : Inport
  LFP cutoff : Inport  Port=2
  LPF zeta : Inport  Port=3
  ConstrolOnOff : Inport  Port=4
  Add5 : Sum  Inputs=+++
  Divide{,1..4} (5 alike) : Product  Inputs=**
  Dot : Subsystem
      mask Display: disp('dot')
  Dot1 : Subsystem
      mask Display: disp('dot')
  Dot2 : Subsystem
      mask Display: disp('dot')
  NominalModel_Kn : Constant  Value=0
  Scope : Scope
      settings: ActiveDisplayYMinimum=-1  ActiveDisplayYMaximum=1  DataLoggingVariableName=ScopeData2
  Scope1 : Scope
      settings: ActiveDisplayYMinimum=-1  ActiveDisplayYMaximum=1  DataLoggingVariableName=ScopeData5
  Second order LPF : Subsystem
  before_dot : Scope
      settings: DataLoggingVariableName=ScopeData3
  commad : Scope
      settings: DataLoggingVariableName=ScopeData4
  FF : Outport  VectorParamsAs1DForOutWhenUnconnected=off
  wires:
  Dot/1(out) -> Dot2/1(in)
  Dot1/1(out) -> Divide1/1
  LFP cutoff/1 -> Second order LPF/2(fc)
  Dot2/1(out) -> Divide/1
  Add5/1 -> Second order LPF/1(In)
  LPF zeta/1 -> Second order LPF/3(zeta)
  Divide/1 -> Scope/1, Add5/1
  Divide1/1 -> Scope1/1, Add5/2
  Divide2/1 -> Add5/3
  [Local_Jn] -> Divide/2
  [Local_Bn] -> Divide1/2
  [Local_Kn] -> Divide2/2
  [steer_Jn] -> [Local_Jn]
  [steer_Bn] -> [Local_Bn]
  NominalModel_Kn/1 -> [Local_Kn]
  Second order LPF/1(Out) -> Divide3/1
  Divide3/1 -> FF/1
  ConstrolOnOff/1 -> Divide4/2, Divide3/2
  Divide4/1 -> Divide2/1, Dot1/1(in), before_dot/1, Dot/1(in)
  command/1 -> commad/1, Divide4/1

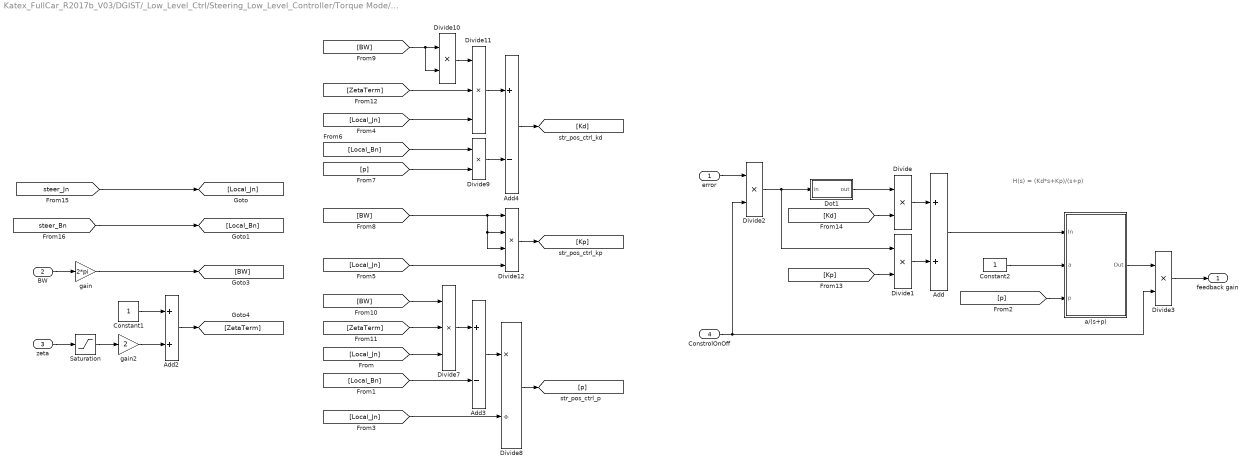
== system Katex_FullCar_R2017b_V03/DGIST/_Low_Level_Ctrl/Steering_Low_Level_Controller/Torque Mode/Steering Motor Control2/Lag compensator(zeta) ==
  note: H(s) = (Kd*s+Kp)/(s+p)
  error : Inport
  BW : Inport  Port=2
  zeta : Inport  Port=3
  ConstrolOnOff : Inport  Port=4
  Add : Sum
  Add2 : Sum
  Add3 : Sum  Inputs=+-
  Add4 : Sum  Inputs=+-
  Constant1 : Constant  SampleTime=Ts
  Constant2 : Constant  SampleTime=Ts
  Divide{,1..3,9..10} (6 alike) : Product  Inputs=**
  Divide11 : Product  Inputs=***
  Divide12 : Product  Inputs=****
  Divide7 : Product  Inputs=***
  Divide8 : Product  Inputs=*/
  Dot1 : Subsystem
      mask Display: disp('dot')
  Saturation : Saturate  UpperLimit=1.5  LowerLimit=0.5
  a/(s+p) : Subsystem
  "gain " : Gain  Gain=2*pi
  gain2 : Gain  Gain=2
  feedback gain : Outport  VectorParamsAs1DForOutWhenUnconnected=off
  wires:
  BW/1 -> "gain "/1
  Add/1 -> a/(s+p)/1(In)
  Divide/1 -> Add/1
  Dot1/1(out) -> Divide/1
  Constant2/1 -> a/(s+p)/2(a)
  zeta/1 -> Saturation/1
  Saturation/1 -> gain2/1
  gain2/1 -> Add2/2
  Constant1/1 -> Add2/1
  [Local_Jn] -> Divide7/3
  Divide7/1 -> Add3/1
  [Local_Bn] -> Add3/2
  Add3/1 -> Divide8/1
  Divide10/1 -> Divide11/1
  Divide8/1 -> [p]
  Divide9/1 -> Add4/2
  Divide11/1 -> Add4/1
  [p] -> a/(s+p)/3(p)
  Divide1/1 -> Add/2
  [Local_Jn] -> Divide8/2
  [Local_Jn] -> Divide11/3
  [Local_Jn] -> Divide12/4
  [Local_Bn] -> Divide9/1
  [p] -> Divide9/2
  "gain "/1 -> [BW]
  [BW] -> Divide12/3, Divide12/2, Divide12/1
  [BW] -> Divide10/2, Divide10/1
  [BW] -> Divide7/1
  Add2/1 -> [ZetaTerm]
  [ZetaTerm] -> Divide7/2
  [ZetaTerm] -> Divide11/2
  Add4/1 -> [Kd]
  Divide12/1 -> [Kp]
  [Kp] -> Divide1/2
  [Kd] -> Divide/2
  [steer_Jn] -> [Local_Jn]
  [steer_Bn] -> [Local_Bn]
  error/1 -> Divide2/1
  Divide2/1 -> Divide1/1, Dot1/1(in)
  ConstrolOnOff/1 -> Divide3/2, Divide2/2
  a/(s+p)/1(Out) -> Divide3/1
  Divide3/1 -> feedback gain/1

== system Katex_FullCar_R2017b_V03/DGIST/_Low_Level_Ctrl/Steering_Low_Level_Controller/Torque Mode/Steering Motor Control2/Poleplacement(PI)1 ==
  note: H(s) = (Kp+Ki)/(s)
  error : Inport
  BW : Inport  Port=2
  zeta : Inport  Port=3
  ConstrolOnOff : Inport  Port=4
  ControlInputError : Inport  Port=5
  Add : Sum
  Add1 : Sum  Inputs=+-
  Constant1 : Constant  Value=Ts
  Divide{,1..5,7} (7 alike) : Product  Inputs=**
  Divide6 : Product  Inputs=***
  Divide9 : Product  Inputs=**/
  Integrator1 : Subsystem
      mask Display: disp('Integator')
  Saturation : Saturate  UpperLimit=3  LowerLimit=0.5
  Saturation Dynamic : simulink/Discontinuities/Saturation Dynamic  OutMin=[]  OutMax=[]  OutDataTypeStr=Inherit: Same as second input  OutDataType=fixdt(1, 16)  OutScaling=2^-10  DoSatur=off
  Sum1 : Sum  Inputs=|++
  Sum2 : Sum  Inputs=++|
  "gain " : Gain  Gain=2*pi
  gain 1 : Gain  Gain=2
  feedback gain : Outport  VectorParamsAs1DForOutWhenUnconnected=off
  wires:
  BW/1 -> "gain "/1
  zeta/1 -> Saturation/1
  Saturation/1 -> gain 1/1
  [Local_Bn] -> Add1/2
  Divide1/1 -> Sum1/1
  Divide2/1 -> Sum1/2
  Integrator1/1(out) -> Divide2/1
  gain 1/1 -> Divide6/1
  Divide3/1 -> Divide4/1
  [Local_Jn] -> Divide4/2
  [Local_Jn] -> Divide6/3
  Divide6/1 -> Add1/1
  Add1/1 -> [Kp]
  Divide4/1 -> [Ki]
  [Kp] -> Divide1/1
  error/1 -> Divide/1
  Sum1/1 -> Divide5/1
  Divide5/1 -> feedback gain/1
  ConstrolOnOff/1 -> Divide5/2, Integrator1/2("Off : 0 On : 1"), Divide/2
  [Ki] -> Divide2/2
  ControlInputError/1 -> Divide7/1
  Divide/1 -> Divide1/2, Sum2/1
  Sum2/1 -> Integrator1/1(in)
  Divide7/1 -> Sum2/2
  Add/1 -> Saturation Dynamic/1
  Divide9/1 -> [AntiWindup]
  Constant1/1 -> Saturation Dynamic/3
  "gain "/1 -> Divide9/2, Add/1, Divide9/1, Divide6/2, Divide3/1, Divide3/2
  [Ki] -> Add/2, Saturation Dynamic/2
  [AntiWindup] -> Divide7/2
  Saturation Dynamic/1 -> Divide9/3
  [steer_Jn] -> [Local_Jn]
  [steer_Bn] -> [Local_Bn]

== system Katex_FullCar_R2017b_V03/DGIST/_Low_Level_Ctrl/Steering_Low_Level_Controller/Torque Mode/Steering Motor Control2/Steering Ref Mode  ==
  Constant2 : Constant  Value=0
  If : If  IfExpression=u1 == 0  ElseIfExpressions=u1 ==1
  If Action Subsystem : Subsystem  TreatAsAtomicUnit=on
  If Action Subsystem1 : Subsystem  TreatAsAtomicUnit=on
  If Action Subsystem2 : Subsystem  TreatAsAtomicUnit=on
  Merge : Merge  Inputs=3
  Out1 : Outport  VectorParamsAs1DForOutWhenUnconnected=off
  wires:
  Constant2/1 -> If Action Subsystem/1(In1)
  [sine_ref] -> If Action Subsystem1/1(In1)
  Merge/1 -> Out1/1
  If Action Subsystem/1(Out1) -> Merge/1
  If Action Subsystem2/1(Out1) -> Merge/3
  [str_load_target_pos] -> If Action Subsystem2/1(In1)
  If Action Subsystem1/1(Out1) -> Merge/2
  If/2 -> If Action Subsystem1/Action
  If/3 -> If Action Subsystem2/Action
  [str_ref_mode] -> If/1
  If/1 -> If Action Subsystem/Action

== system Katex_FullCar_R2017b_V03/DGIST/_Low_Level_Ctrl/Steering_Low_Level_Controller/Torque Mode/Steering Motor Control2/Steering system ==
  note: mN*m
  note: Motor N*m
  note: Load N*m
  N*m : Inport
  Constant : Constant  Value=55.08
  Constant1 : Constant  Value=1000
  Constant2 : Constant  Value=315
  Divide : Product  Inputs=*/
  Divide1 : Product  Inputs=**
  Divide3 : Product  Inputs=*/
  Gain : Gain  Gain=1000
  Gain1 : Gain  Gain=-1
  Saturation Dynamic : simulink/Discontinuities/Saturation Dynamic  OutMin=[]  OutMax=[]  OutDataTypeStr=Inherit: Same as second input  OutDataType=fixdt(1, 16)  OutScaling=2^-10  DoSatur=off
  Target Torque : Outport  VectorParamsAs1DForOutWhenUnconnected=off
  tag scope: closed_ID_FB=global
  wires:
  Constant2/1 -> Divide3/2
  Gain/1 -> Target Torque/1
  Divide/1 -> Gain/1
  N*m/1 -> Divide3/1
  Divide1/1 -> [closed_ID_FB], Saturation Dynamic/2
  Constant1/1 -> Divide1/2
  Divide3/1 -> Divide1/1
  Saturation Dynamic/1 -> Divide/1
  Gain1/1 -> Saturation Dynamic/3
  Constant/1 -> Saturation Dynamic/1, Gain1/1, Divide/2

== system Katex_FullCar_R2017b_V03/DGIST/_Low_Level_Ctrl/Steering_Low_Level_Controller/Torque Mode/Steering Motor Control2/Steering system1 ==
  note: mN*m
  note: Motor N*m
  note: Load N*m
  N*m : Inport
  Constant1 : Constant  Value=1000
  Constant2 : Constant  Value=315
  Divide : Product  Inputs=*/
  Divide1 : Product  Inputs=**
  Divide3 : Product  Inputs=*/
  Gain : Gain  Gain=1000
  Gain1 : Gain  Gain=-1
  Saturation Dynamic : sl_discontinuities/Saturation Dynamic  OutMin=[]  OutMax=[]  OutDataTypeStr=Inherit: Same as second input  OutDataType=fixdt(1, 16)  OutScaling=2^-10  DoSatur=off
  Target Torque : Outport  VectorParamsAs1DForOutWhenUnconnected=off
  wires:
  Constant2/1 -> Divide3/2
  Gain/1 -> Target Torque/1
  Divide/1 -> Gain/1
  N*m/1 -> Divide3/1
  Divide1/1 -> Saturation Dynamic/2
  Constant1/1 -> Divide1/2
  Divide3/1 -> Divide1/1
  Saturation Dynamic/1 -> Divide/1
  Gain1/1 -> Saturation Dynamic/3
  [str_rated_torque] -> Saturation Dynamic/1, Gain1/1, Divide/2

== system Katex_FullCar_R2017b_V03/DGIST/_Low_Level_Ctrl/Steering_Low_Level_Controller/Torque Mode/Steering Motor Control3/DOB(theta) ==
  U_in*(Tm) : Inport
  Y_out(theta) : Inport  Port=2
  CutoffFreq_Q : Inport  Port=3
  ConstrolOnOff : Inport  Port=4
  Add1 : Sum  Inputs=-+
  Add5 : Sum  Inputs=+++
  Delay : Delay  DelayLength=1  InitialCondition=0
  Divide{,1..5} (6 alike) : Product  Inputs=**
  Dot : Subsystem
      mask Display: disp('dot')
  Dot1 : Subsystem
      mask Display: disp('dot')
  Dot2 : Subsystem
      mask Display: disp('dot')
  NominalModel_Kn : Constant  Value=0
  Scope1 : Scope
  Scope2 : Scope
      settings: DataLoggingVariableName=ScopeData2
  Scope3 : Scope
      settings: DataLoggingVariableName=ScopeData3
  Second order LPF : Subsystem
  zeta : Constant  SampleTime=Ts
  Dist_hat : Outport  VectorParamsAs1DForOutWhenUnconnected=off
  wires:
  Add5/1 -> Add1/2
  CutoffFreq_Q/1 -> Second order LPF/2(fc)
  zeta/1 -> Second order LPF/3(zeta)
  [steer_Jn] -> [Local_Jn]
  NominalModel_Kn/1 -> [Local_Kn]
  [steer_Bn] -> [Local_Bn]
  Y_out(theta)/1 -> Scope1/1, Divide4/1
  [Local_Jn] -> Divide/2
  [Local_Kn] -> Divide2/2
  Dot1/1(out) -> Divide1/1
  [Local_Bn] -> Divide1/2
  Dot/1(out) -> Dot2/1(in)
  Divide/1 -> Add5/1
  Divide2/1 -> Add5/3
  Divide1/1 -> Add5/2
  Dot2/1(out) -> Divide/1
  ConstrolOnOff/1 -> Divide5/2, Divide3/2, Divide4/2
  Divide4/1 -> Divide2/1, Dot1/1(in), Dot/1(in)
  U_in*(Tm)/1 -> Delay/1
  Divide3/1 -> Add1/1
  Second order LPF/1(Dist_hat) -> Divide5/1
  Divide5/1 -> Scope2/1, Dist_hat/1
  Delay/1 -> Divide3/1
  Add1/1 -> Scope3/1, Second order LPF/1(In)

== system Katex_FullCar_R2017b_V03/DGIST/_Low_Level_Ctrl/Steering_Low_Level_Controller/Torque Mode/Steering Motor Control3/Feedforward(theta) ==
  command : Inport
  LFP cutoff : Inport  Port=2
  LPF zeta : Inport  Port=3
  ConstrolOnOff : Inport  Port=4
  Add5 : Sum  Inputs=+++
  Divide{,1..4} (5 alike) : Product  Inputs=**
  Dot : Subsystem
      mask Display: disp('dot')
  Dot1 : Subsystem
      mask Display: disp('dot')
  Dot2 : Subsystem
      mask Display: disp('dot')
  NominalModel_Kn : Constant  Value=0
  Scope : Scope
      settings: ActiveDisplayYMinimum=-1  ActiveDisplayYMaximum=1  DataLoggingVariableName=ScopeData2
  Scope1 : Scope
      settings: ActiveDisplayYMinimum=-1  ActiveDisplayYMaximum=1  DataLoggingVariableName=ScopeData5
  Second order LPF : Subsystem
  before_dot : Scope
      settings: DataLoggingVariableName=ScopeData3
  commad : Scope
      settings: DataLoggingVariableName=ScopeData4
  FF : Outport  VectorParamsAs1DForOutWhenUnconnected=off
  wires:
  Dot/1(out) -> Dot2/1(in)
  Dot1/1(out) -> Divide1/1
  LFP cutoff/1 -> Second order LPF/2(fc)
  Dot2/1(out) -> Divide/1
  Add5/1 -> Second order LPF/1(In)
  LPF zeta/1 -> Second order LPF/3(zeta)
  Divide/1 -> Scope/1, Add5/1
  Divide1/1 -> Scope1/1, Add5/2
  Divide2/1 -> Add5/3
  [Local_Jn] -> Divide/2
  [Local_Bn] -> Divide1/2
  [Local_Kn] -> Divide2/2
  [steer_Jn] -> [Local_Jn]
  [steer_Bn] -> [Local_Bn]
  NominalModel_Kn/1 -> [Local_Kn]
  Second order LPF/1(Out) -> Divide3/1
  Divide3/1 -> FF/1
  ConstrolOnOff/1 -> Divide4/2, Divide3/2
  Divide4/1 -> Divide2/1, Dot1/1(in), before_dot/1, Dot/1(in)
  command/1 -> commad/1, Divide4/1

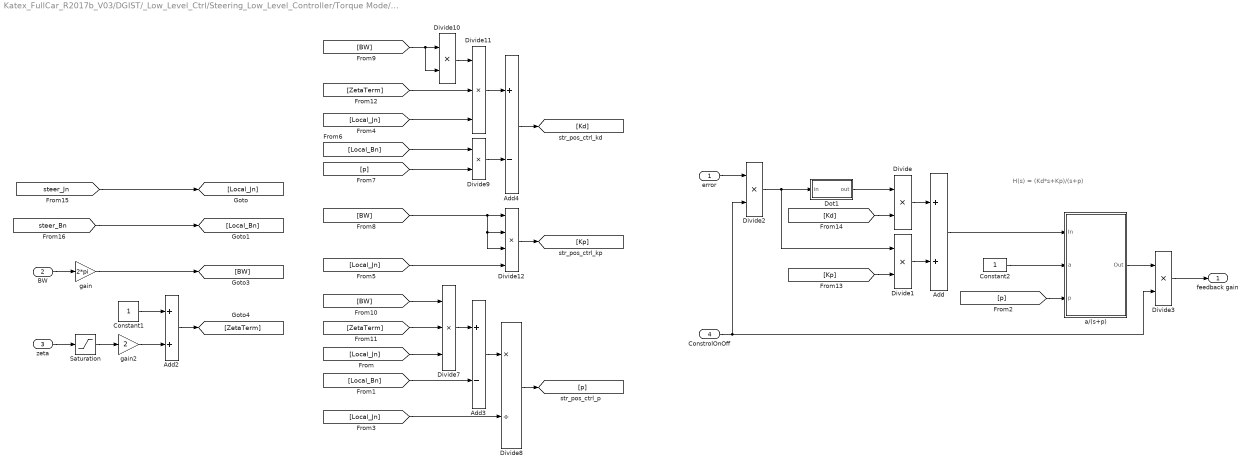
== system Katex_FullCar_R2017b_V03/DGIST/_Low_Level_Ctrl/Steering_Low_Level_Controller/Torque Mode/Steering Motor Control3/Lag compensator(zeta) ==
  note: H(s) = (Kd*s+Kp)/(s+p)
  error : Inport
  BW : Inport  Port=2
  zeta : Inport  Port=3
  ConstrolOnOff : Inport  Port=4
  Add : Sum
  Add2 : Sum
  Add3 : Sum  Inputs=+-
  Add4 : Sum  Inputs=+-
  Constant1 : Constant  SampleTime=Ts
  Constant2 : Constant  SampleTime=Ts
  Divide{,1..3,9..10} (6 alike) : Product  Inputs=**
  Divide11 : Product  Inputs=***
  Divide12 : Product  Inputs=****
  Divide7 : Product  Inputs=***
  Divide8 : Product  Inputs=*/
  Dot1 : Subsystem
      mask Display: disp('dot')
  Saturation : Saturate  UpperLimit=1.5  LowerLimit=0.5
  a/(s+p) : Subsystem
  "gain " : Gain  Gain=2*pi
  gain2 : Gain  Gain=2
  feedback gain : Outport  VectorParamsAs1DForOutWhenUnconnected=off
  wires:
  BW/1 -> "gain "/1
  Add/1 -> a/(s+p)/1(In)
  Divide/1 -> Add/1
  Dot1/1(out) -> Divide/1
  Constant2/1 -> a/(s+p)/2(a)
  zeta/1 -> Saturation/1
  Saturation/1 -> gain2/1
  gain2/1 -> Add2/2
  Constant1/1 -> Add2/1
  [Local_Jn] -> Divide7/3
  Divide7/1 -> Add3/1
  [Local_Bn] -> Add3/2
  Add3/1 -> Divide8/1
  Divide10/1 -> Divide11/1
  Divide8/1 -> [p]
  Divide9/1 -> Add4/2
  Divide11/1 -> Add4/1
  [p] -> a/(s+p)/3(p)
  Divide1/1 -> Add/2
  [Local_Jn] -> Divide8/2
  [Local_Jn] -> Divide11/3
  [Local_Jn] -> Divide12/4
  [Local_Bn] -> Divide9/1
  [p] -> Divide9/2
  "gain "/1 -> [BW]
  [BW] -> Divide12/3, Divide12/2, Divide12/1
  [BW] -> Divide10/2, Divide10/1
  [BW] -> Divide7/1
  Add2/1 -> [ZetaTerm]
  [ZetaTerm] -> Divide7/2
  [ZetaTerm] -> Divide11/2
  Add4/1 -> [Kd]
  Divide12/1 -> [Kp]
  [Kp] -> Divide1/2
  [Kd] -> Divide/2
  [steer_Jn] -> [Local_Jn]
  [steer_Bn] -> [Local_Bn]
  error/1 -> Divide2/1
  Divide2/1 -> Divide1/1, Dot1/1(in)
  ConstrolOnOff/1 -> Divide3/2, Divide2/2
  a/(s+p)/1(Out) -> Divide3/1
  Divide3/1 -> feedback gain/1

== system Katex_FullCar_R2017b_V03/DGIST/_Low_Level_Ctrl/Steering_Low_Level_Controller/Torque Mode/Steering Motor Control3/Steering system1 ==
  note: mN*m
  note: Motor N*m
  note: Load N*m
  N*m : Inport
  Constant1 : Constant  Value=1000
  Constant2 : Constant  Value=315
  Divide : Product  Inputs=*/
  Divide1 : Product  Inputs=**
  Divide3 : Product  Inputs=*/
  Gain : Gain  Gain=1000
  Gain1 : Gain  Gain=-1
  Saturation Dynamic : sl_discontinuities/Saturation Dynamic  OutMin=[]  OutMax=[]  OutDataTypeStr=Inherit: Same as second input  OutDataType=fixdt(1, 16)  OutScaling=2^-10  DoSatur=off
  Target Torque : Outport  VectorParamsAs1DForOutWhenUnconnected=off
  wires:
  Constant2/1 -> Divide3/2
  Gain/1 -> Target Torque/1
  Divide/1 -> Gain/1
  N*m/1 -> Divide3/1
  Divide1/1 -> Saturation Dynamic/2
  Constant1/1 -> Divide1/2
  Divide3/1 -> Divide1/1
  Saturation Dynamic/1 -> Divide/1
  Gain1/1 -> Saturation Dynamic/3
  [str_rated_torque] -> Saturation Dynamic/1, Gain1/1, Divide/2

== system Katex_FullCar_R2017b_V03/DGIST/_Low_Level_Ctrl/Suspension_Low_Level_Controller/Torque Mode/Subsystem/DOB(theta) ==
  U_in*(Tm) : Inport
  Y_out(theta) : Inport  Port=2
  CutoffFreq_Q : Inport  Port=3
  ConstrolOnOff : Inport  Port=4
  Add1 : Sum  Inputs=-+
  Add5 : Sum  Inputs=+++
  Delay : Delay  DelayLength=1  InitialCondition=0
  Divide{,1..5} (6 alike) : Product  Inputs=**
  Dot : Subsystem
      mask Display: disp('dot')
  Dot1 : Subsystem
      mask Display: disp('dot')
  Dot2 : Subsystem
      mask Display: disp('dot')
  NominalModel_Kn : Constant  Value=0
  Scope1 : Scope
  Scope2 : Scope
      settings: DataLoggingVariableName=ScopeData2
  Scope3 : Scope
      settings: DataLoggingVariableName=ScopeData3
  Second order LPF : Subsystem
  zeta : Constant  SampleTime=Ts
  Dist_hat : Outport  VectorParamsAs1DForOutWhenUnconnected=off
  wires:
  Add5/1 -> Add1/2
  CutoffFreq_Q/1 -> Second order LPF/2(fc)
  zeta/1 -> Second order LPF/3(zeta)
  [sus_Jn] -> [Local_Jn]
  NominalModel_Kn/1 -> [Local_Kn]
  [sus_Bn] -> [Local_Bn]
  Y_out(theta)/1 -> Scope1/1, Divide4/1
  [Local_Jn] -> Divide/2
  [Local_Kn] -> Divide2/2
  Dot1/1(out) -> Divide1/1
  [Local_Bn] -> Divide1/2
  Dot/1(out) -> Dot2/1(in)
  Divide/1 -> Add5/1
  Divide2/1 -> Add5/3
  Divide1/1 -> Add5/2
  Dot2/1(out) -> Divide/1
  ConstrolOnOff/1 -> Divide5/2, Divide3/2, Divide4/2
  Divide4/1 -> Divide2/1, Dot1/1(in), Dot/1(in)
  U_in*(Tm)/1 -> Delay/1
  Divide3/1 -> Add1/1
  Second order LPF/1(Dist_hat) -> Divide5/1
  Divide5/1 -> Scope2/1, Dist_hat/1
  Delay/1 -> Divide3/1
  Add1/1 -> Scope3/1, Second order LPF/1(In)

== system Katex_FullCar_R2017b_V03/DGIST/_Low_Level_Ctrl/Suspension_Low_Level_Controller/Torque Mode/Subsystem/Feedforward(theta) ==
  command : Inport
  LFP cutoff : Inport  Port=2
  LPF zeta : Inport  Port=3
  ConstrolOnOff : Inport  Port=4
  Add5 : Sum  Inputs=+++
  Divide{,1..4} (5 alike) : Product  Inputs=**
  Dot : Subsystem
      mask Display: disp('dot')
  Dot1 : Subsystem
      mask Display: disp('dot')
  Dot2 : Subsystem
      mask Display: disp('dot')
  NominalModel_Kn : Constant  Value=0
  Second order LPF : Subsystem
  FF : Outport  VectorParamsAs1DForOutWhenUnconnected=off
  wires:
  Dot/1(out) -> Dot2/1(in)
  Dot1/1(out) -> Divide1/1
  LFP cutoff/1 -> Second order LPF/2(fc)
  Dot2/1(out) -> Divide/1
  Add5/1 -> Second order LPF/1(In)
  LPF zeta/1 -> Second order LPF/3(zeta)
  Divide/1 -> Add5/1
  Divide1/1 -> Add5/2
  Divide2/1 -> Add5/3
  [Local_Jn] -> Divide/2
  [Local_Bn] -> Divide1/2
  [Local_Kn] -> Divide2/2
  [sus_Jn] -> [Local_Jn]
  [sus_Bn] -> [Local_Bn]
  NominalModel_Kn/1 -> [Local_Kn]
  Second order LPF/1(Out) -> Divide3/1
  Divide3/1 -> FF/1
  ConstrolOnOff/1 -> Divide4/2, Divide3/2
  Divide4/1 -> Divide2/1, Dot1/1(in), Dot/1(in)
  command/1 -> Divide4/1

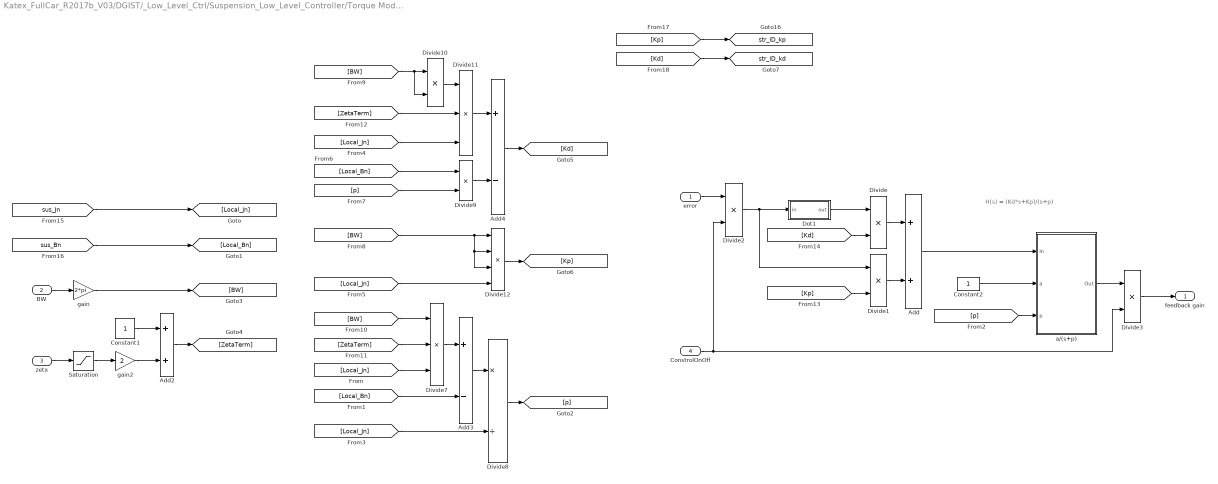
== system Katex_FullCar_R2017b_V03/DGIST/_Low_Level_Ctrl/Suspension_Low_Level_Controller/Torque Mode/Subsystem/Lag compensator(zeta) ==
  note: H(s) = (Kd*s+Kp)/(s+p)
  error : Inport
  BW : Inport  Port=2
  zeta : Inport  Port=3
  ConstrolOnOff : Inport  Port=4
  Add : Sum
  Add2 : Sum
  Add3 : Sum  Inputs=+-
  Add4 : Sum  Inputs=+-
  Constant1 : Constant  SampleTime=Ts
  Constant2 : Constant  SampleTime=Ts
  Divide{,1..3,9..10} (6 alike) : Product  Inputs=**
  Divide11 : Product  Inputs=***
  Divide12 : Product  Inputs=****
  Divide7 : Product  Inputs=***
  Divide8 : Product  Inputs=*/
  Dot1 : Subsystem
      mask Display: disp('dot')
  Saturation : Saturate  UpperLimit=1.5  LowerLimit=0.5
  a/(s+p) : Subsystem
  "gain " : Gain  Gain=2*pi
  gain2 : Gain  Gain=2
  feedback gain : Outport  VectorParamsAs1DForOutWhenUnconnected=off
  tag scope: str_ID_kd=global, str_ID_kp=global
  wires:
  BW/1 -> "gain "/1
  Add/1 -> a/(s+p)/1(In)
  Divide/1 -> Add/1
  Dot1/1(out) -> Divide/1
  Constant2/1 -> a/(s+p)/2(a)
  zeta/1 -> Saturation/1
  Saturation/1 -> gain2/1
  gain2/1 -> Add2/2
  Constant1/1 -> Add2/1
  [Local_Jn] -> Divide7/3
  Divide7/1 -> Add3/1
  [Local_Bn] -> Add3/2
  Add3/1 -> Divide8/1
  Divide10/1 -> Divide11/1
  Divide8/1 -> [p]
  Divide9/1 -> Add4/2
  Divide11/1 -> Add4/1
  [p] -> a/(s+p)/3(p)
  Divide1/1 -> Add/2
  [Local_Jn] -> Divide8/2
  [Local_Jn] -> Divide11/3
  [Local_Jn] -> Divide12/4
  [Local_Bn] -> Divide9/1
  [p] -> Divide9/2
  "gain "/1 -> [BW]
  [BW] -> Divide12/3, Divide12/2, Divide12/1
  [BW] -> Divide10/2, Divide10/1
  [BW] -> Divide7/1
  Add2/1 -> [ZetaTerm]
  [ZetaTerm] -> Divide7/2
  [ZetaTerm] -> Divide11/2
  Add4/1 -> [Kd]
  Divide12/1 -> [Kp]
  [Kp] -> Divide1/2
  [Kd] -> Divide/2
  [sus_Jn] -> [Local_Jn]
  [sus_Bn] -> [Local_Bn]
  error/1 -> Divide2/1
  Divide2/1 -> Divide1/1, Dot1/1(in)
  ConstrolOnOff/1 -> Divide3/2, Divide2/2
  a/(s+p)/1(Out) -> Divide3/1
  Divide3/1 -> feedback gain/1
  [Kp] -> [str_ID_kp]
  [Kd] -> [str_ID_kd]

== system Katex_FullCar_R2017b_V03/DGIST/_Low_Level_Ctrl/Suspension_Low_Level_Controller/Torque Mode/Subsystem/Sus Ref Mode ==
  Constant2 : Constant  Value=0
  If : If  IfExpression=u1 == 0  ElseIfExpressions=u1 ==1
  If Action Subsystem : Subsystem  TreatAsAtomicUnit=on
  If Action Subsystem1 : Subsystem  TreatAsAtomicUnit=on
  If Action Subsystem2 : Subsystem  TreatAsAtomicUnit=on
  Merge : Merge  Inputs=3
  Out1 : Outport  VectorParamsAs1DForOutWhenUnconnected=off
  wires:
  Constant2/1 -> If Action Subsystem/1(In1)
  [sine_ref] -> If Action Subsystem1/1(In1)
  Merge/1 -> Out1/1
  If Action Subsystem/1(Out1) -> Merge/1
  If Action Subsystem2/1(Out1) -> Merge/3
  [sus_load_target_pos] -> If Action Subsystem2/1(In1)
  If Action Subsystem1/1(Out1) -> Merge/2
  If/2 -> If Action Subsystem1/Action
  If/3 -> If Action Subsystem2/Action
  [sus_ref_mode] -> If/1
  If/1 -> If Action Subsystem/Action

== system Katex_FullCar_R2017b_V03/DGIST/_Low_Level_Ctrl/Suspension_Low_Level_Controller/Torque Mode/Subsystem/Suspension system1 ==
  note: mN*m
  note: Motor N*m
  note: Load N*m
  N*m : Inport
  Constant1 : Constant  Value=1000
  Divide : Product  Inputs=*/
  Divide1 : Product  Inputs=**
  Divide3 : Product  Inputs=*/
  Gain : Gain  Gain=1000
  Gain1 : Gain  Gain=-1
  Saturation Dynamic : sl_discontinuities/Saturation Dynamic  OutMin=[]  OutMax=[]  OutDataTypeStr=Inherit: Same as second input  OutDataType=fixdt(1, 16)  OutScaling=2^-10  DoSatur=off
  Target Torque : Outport  VectorParamsAs1DForOutWhenUnconnected=off
  tag scope: For_ID_control_torque_sus=global
  wires:
  [N_sus] -> Divide3/2
  Gain/1 -> Target Torque/1
  Divide/1 -> Gain/1
  N*m/1 -> Divide3/1
  Divide1/1 -> Saturation Dynamic/2
  Constant1/1 -> Divide1/2
  Divide3/1 -> [For_ID_control_torque_sus], Divide1/1
  Saturation Dynamic/1 -> Divide/1
  Gain1/1 -> Saturation Dynamic/3
  [sus_rated_torque] -> Saturation Dynamic/1, Gain1/1, Divide/2
